simulink model "project1"  (R2020b)
settings: Solver=VariableStepAuto  StartTime=0.0  StopTime=10.0  RelTol=1e-3
settings Model: Creator=sushma  LastModifiedBy=sushma

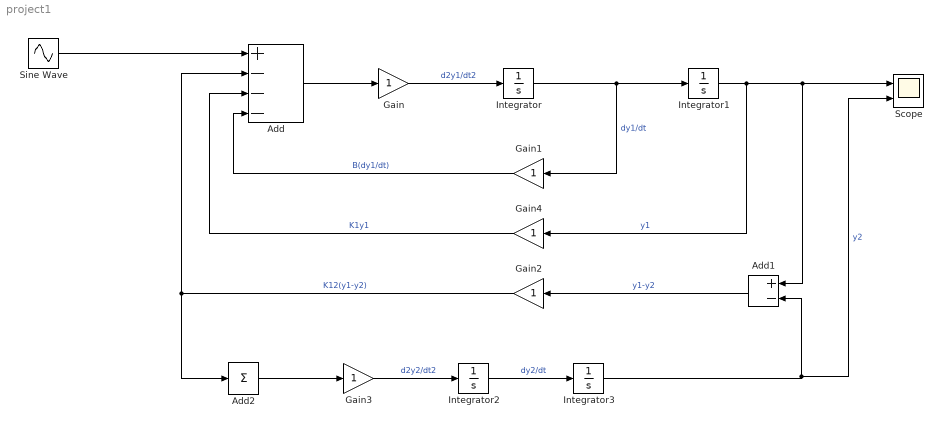
== system project1 ==
  Add : Sum  Inputs=+---
  Add1 : Sum  Inputs=+-
  Add2 : Sum  Inputs=+
  Gain{,1..4} (5 alike) : Gain
  Integrator{,1..3} (4 alike) : Integrator
  Scope : Scope  NumInputPorts=2
  Sine Wave : Sin  Amplitude=2  Frequency=10  SampleTime=0
  wires:
  Add2/1 -> Gain3/1
  Gain2/1 -> Add2/1, Add/2  "K12(y1-y2)"
  Gain3/1 -> Integrator2/1  "d2y2/dt2"
  Gain1/1 -> Add/4  "B(dy1/dt)"
  Gain/1 -> Integrator/1  "d2y1/dt2"
  Integrator1/1 -> Gain4/1, Scope/1, Add1/1  "y1"
  Gain4/1 -> Add/3  "K1y1"
  Integrator3/1 -> Scope/2, Add1/2  "y2"
  Add1/1 -> Gain2/1  "y1-y2"
  Integrator2/1 -> Integrator3/1  "dy2/dt"
  Add/1 -> Gain/1
  Sine Wave/1 -> Add/1
  Integrator/1 -> Gain1/1, Integrator1/1  "dy1/dt"
